simulink model "bi_real_unscr_4x_plan"  (Simulink 7.6)
settings: Solver=ode45  StartTime=0.0  StopTime=10.0  RelTol=1e-3
undefined symbols (not defined in the file or in its folder): add_latency
libraries: xbsIndex_r4 x259, casper_library x9, monroe_library x3
(part 1 of 2)
settings Model: Creator=monroe  LastModifiedBy=Ryan

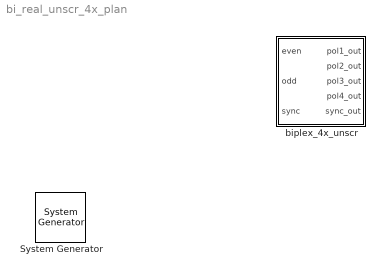
== system bi_real_unscr_4x_plan ==
  " System Generator" : xbsIndex_r4/ System Generator  Tag=genX  SystemSampleTime=-1  xilinxfamily=Virtex6  part=xc6vsx315t  speed=-3  package=ff1156  synthesis_tool=XST  clock_wrapper=Clock Enables  directory=./netlist  testbench=off  simulink_period=1  sysclk_period=10  dcm_input_clock_period=10  incr_netlist=off  trim_vbits=Everywhere in SubSystem  dbl_ovrd=According to Block Masks  core_generation=According to Block Masks  run_coregen=off  deprecated_control=off  eval_field=0  block_type=sysgen
  biplex_4x_unscr : Subsystem  mask{FFTSize=10, bram_latency=3, input_bit_width=18, reorder_din_latency=0}
      mask prompts: FFTSize "Size of FFT (2^?):"; bram_latency "BRAM Latency"; input_bit_width "Input Bit Width"; reorder_din_latency "Reorder Data In Latency"

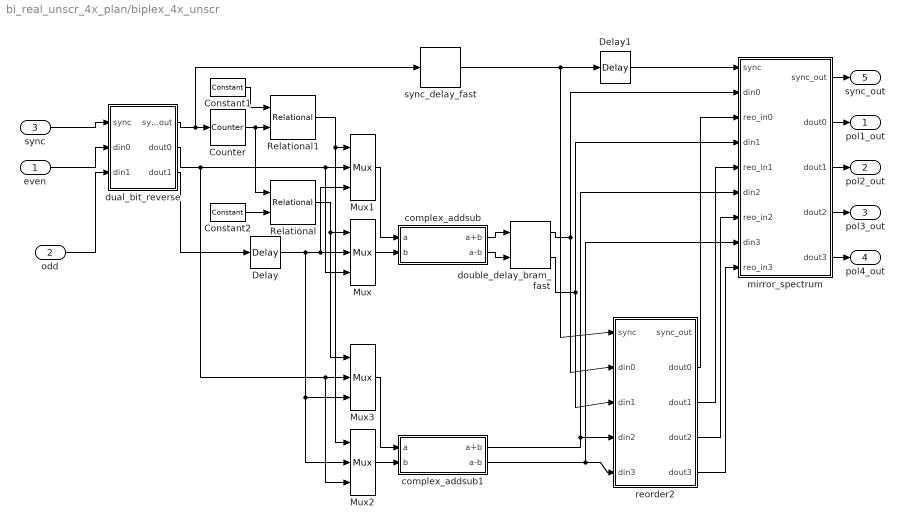
== system bi_real_unscr_4x_plan/biplex_4x_unscr ==
  even : Inport
  odd : Inport  Port=2
  sync : Inport  Port=3
  Constant1 : xbsIndex_r4/Constant  arith_type=Unsigned  const=2^(FFTSize-1)-1  n_bits=FFTSize  bin_pt=0  explicit_period=on  period=1  equ=P=C  opselect=C  inp2=PCIN>>17  opr=+  inp1=P  carry=CIN  dbl_ovrd=off  block_type=constant
      settings: block_version=9.1.01
  Constant2 : xbsIndex_r4/Constant  arith_type=Unsigned  const=2^FFTSize -1  n_bits=FFTSize  bin_pt=0  explicit_period=on  period=1  equ=P=C  opselect=C  inp2=PCIN>>17  opr=+  inp1=P  carry=CIN  dbl_ovrd=off  block_type=constant
      settings: block_version=9.1.01
  Counter : xbsIndex_r4/Counter  cnt_type=Free Running  cnt_to=Inf  operation=Up  start_count=0  cnt_by_val=1  arith_type=Unsigned  n_bits=FFTSize  bin_pt=0  load_pin=off  rst=on  en=off  explicit_period=off  period=1  dbl_ovrd=off  use_behavioral_HDL=off  implementation=Fabric  use_rpm=on  block_type=counter
      settings: xl_area=[0, 0, 0, 0, 0, 0, 0]  block_version=9.1.01
  Delay : xbsIndex_r4/Delay  en=off  latency=1  dbl_ovrd=off  reg_retiming=off  block_type=delay
      settings: xl_area=[0, 0, 0, 0, 0, 0, 0]  block_version=9.1.01
  Delay1 : xbsIndex_r4/Delay  en=off  latency=3  dbl_ovrd=off  reg_retiming=off  block_type=delay
      settings: xl_area=[0, 0, 0, 0, 0, 0, 0]  block_version=9.1.01
  Mux{,1..3} (4 alike) : xbsIndex_r4/Mux  inputs=2  en=off  latency=1  precision=Full  arith_type="Signed  (2's comp)"  n_bits=8  bin_pt=2  quantization=Truncate  overflow=Wrap  dbl_ovrd=off  block_type=mux
      settings: xl_area=[0, 0, 0, 0, 0, 0, 0]  block_version=9.1.01
  Relational : xbsIndex_r4/Relational  mode=a=b  en=off  latency=1  dbl_ovrd=off  block_type=relational
      settings: xl_area=[0, 0, 0, 0, 0, 0, 0]  block_version=9.1.01
  Relational1 : xbsIndex_r4/Relational  mode=a=b  en=off  latency=1  dbl_ovrd=off  block_type=relational
      settings: xl_area=[0, 0, 0, 0, 0, 0, 0]  block_version=9.1.01
  complex_addsub : Subsystem  mask(complex_addsub){BitWidth=input_bit_width, add_latency=add_latency}
      mask prompts: BitWidth "Bit Wdith"; add_latency "Add Latency"
      mask help:
      | Adds and subtracts the complex inputs.
      | If a = w + ix, b = y + iz then
      | a+b = (w+y)/2 + i(x-z)/2 and
      | a-b = (x+z)/2 + i(y-w)/2
  complex_addsub1 : Subsystem  mask(complex_addsub){BitWidth=input_bit_width, add_latency=add_latency}
      mask prompts: BitWidth "Bit Wdith"; add_latency "Add Latency"
      mask help:
      | Adds and subtracts the complex inputs.
      | If a = w + ix, b = y + iz then
      | a+b = (w+y)/2 + i(x-z)/2 and
      | a-b = (x+z)/2 + i(y-w)/2
  double_delay_bram_fast : monroe_library/double_delay_bram_fast  SystemSampleTime=-1  delay_len=2^(FFTSize-1)  bram_latency=bram_latency
  dual_bit_reverse : Subsystem  AncestorBlock=casper_library/Reorder/reorder  mask(reorder){bram_latency=bram_latency, din_latency=reorder_din_latency}
      mask prompts: bram_latency "BRAM Latency"; din_latency "Data In Latency"
      settings: AttributesFormatString=order=2
  mirror_spectrum : Subsystem
  reorder2 : Subsystem  AncestorBlock=casper_library/Reorder/reorder  mask(reorder){bram_latency=bram_latency, din_delay=1, map_latency=0, din_bit_width=input_bit_width}
      mask prompts: bram_latency "BRAM Latency"; din_delay "Data In Delay"; map_latency "Map Latency"; din_bit_width "Data In Bit Width"
      settings: AttributesFormatString=order=2
  sync_delay_fast : monroe_library/sync_delay_fast  SystemSampleTime=-1  delay_len=2^(FFTSize-1)+2
  pol1_out : Outport
  pol2_out : Outport  Port=2
  pol3_out : Outport  Port=3
  pol4_out : Outport  Port=4
  sync_out : Outport  Port=5
  wires:
  Delay1/1 -> mirror_spectrum/1(sync)
  mirror_spectrum/5(dout3) -> pol4_out/1
  mirror_spectrum/4(dout2) -> pol3_out/1
  mirror_spectrum/3(dout1) -> pol2_out/1
  odd/1 -> dual_bit_reverse/3(din1)
  even/1 -> dual_bit_reverse/2(din0)
  Relational/1 -> Mux3/1, Mux/1
  Mux/1 -> complex_addsub/2(b)
  Delay/1 -> Mux2/2, Mux3/3, Mux/2, Mux1/3
  dual_bit_reverse/1(sync_out) -> Counter/1, sync_delay_fast/1
  dual_bit_reverse/2(dout0) -> Mux/3, Mux1/2, Mux2/3, Mux3/2
  dual_bit_reverse/3(dout1) -> Delay/1
  sync/1 -> dual_bit_reverse/1(sync)
  Mux1/1 -> complex_addsub/1(a)
  Constant2/1 -> Relational/2
  Counter/1 -> Relational/1, Relational1/2
  Constant1/1 -> Relational1/1
  Relational1/1 -> Mux2/1, Mux1/1
  Mux2/1 -> complex_addsub1/2(b)
  Mux3/1 -> complex_addsub1/1(a)
  complex_addsub/1(a+b) -> double_delay_bram_fast/1
  complex_addsub/2(a-b) -> double_delay_bram_fast/2
  complex_addsub1/2(a-b) -> reorder2/5(din3), mirror_spectrum/8(din3)
  complex_addsub1/1(a+b) -> reorder2/4(din2), mirror_spectrum/6(din2)
  double_delay_bram_fast/2 -> reorder2/3(din1), mirror_spectrum/4(din1)
  double_delay_bram_fast/1 -> reorder2/2(din0), mirror_spectrum/2(din0)
  sync_delay_fast/1 -> Delay1/1, reorder2/1(sync)
  mirror_spectrum/1(sync_out) -> sync_out/1
  mirror_spectrum/2(dout0) -> pol1_out/1
  reorder2/3(dout1) -> mirror_spectrum/5(reo_in1)
  reorder2/2(dout0) -> mirror_spectrum/3(reo_in0)
  reorder2/4(dout2) -> mirror_spectrum/7(reo_in2)
  reorder2/5(dout3) -> mirror_spectrum/9(reo_in3)

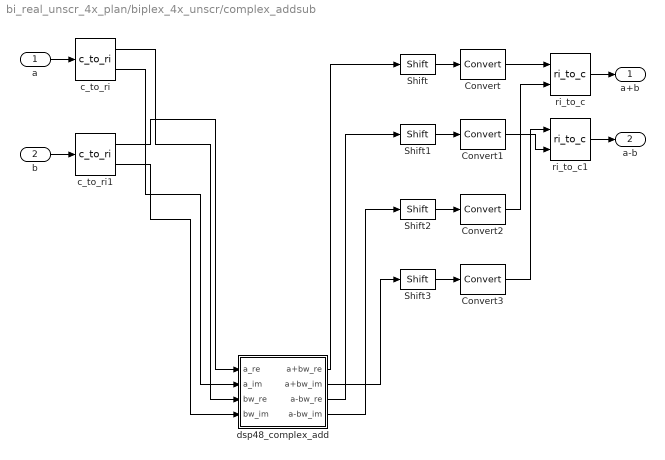
== system bi_real_unscr_4x_plan/biplex_4x_unscr/complex_addsub ==
  a : Inport
  b : Inport  Port=2
  Convert{,1..3} (4 alike) : xbsIndex_r4/Convert  arith_type="Signed  (2's comp)"  n_bits=BitWidth  bin_pt=BitWidth - 1  quantization=Truncate  overflow=Wrap  en=off  latency=add_latency  dbl_ovrd=off  pipeline=off  block_type=convert
      settings: xl_area=[0, 0, 0, 0, 0, 0, 0]
  Shift{,1..3} (4 alike) : xbsIndex_r4/Shift  shift_dir=Right  shift_bits=1  en=off  latency=0  precision=Full  arith_type="Signed  (2's comp)"  n_bits=8  bin_pt=2  quantization=Truncate  overflow=Wrap  dbl_ovrd=off  block_type=shift
      settings: xl_area=[0, 0, 0, 0, 0, 0, 0]  block_version=9.1.01
  c_to_ri : casper_library/Misc/c_to_ri  SystemSampleTime=-1  n_bits=BitWidth  bin_pt=BitWidth-1
      settings: AttributesFormatString=18_17 r/i
  c_to_ri1 : casper_library/Misc/c_to_ri  SystemSampleTime=-1  n_bits=BitWidth  bin_pt=BitWidth-1
      settings: AttributesFormatString=18_17 r/i
  dsp48_complex_add : Subsystem  mask{a_bit_width=BitWidth, a_bin_pt=BitWidth-2, bw_bit_width=BitWidth, bw_bin_pt=BitWidth-2}
      mask prompts: a_bit_width "'a' bit width"; a_bin_pt "'a' binary point"; bw_bit_width "'bw' bit width"; bw_bin_pt "'bw' binary point"
  ri_to_c : casper_library/Misc/ri_to_c  SystemSampleTime=-1
  ri_to_c1 : casper_library/Misc/ri_to_c  SystemSampleTime=-1
  a+b : Outport
  a-b : Outport  Port=2
  wires:
  Convert3/1 -> ri_to_c1/1
  Convert1/1 -> ri_to_c1/2
  c_to_ri/1 -> dsp48_complex_add/3(bw_re)
  c_to_ri/2 -> dsp48_complex_add/2(a_im)
  c_to_ri1/1 -> dsp48_complex_add/1(a_re)
  c_to_ri1/2 -> dsp48_complex_add/4(bw_im)
  Convert/1 -> ri_to_c/1
  Convert2/1 -> ri_to_c/2
  a/1 -> c_to_ri/1
  ri_to_c/1 -> a+b/1
  ri_to_c1/1 -> a-b/1
  b/1 -> c_to_ri1/1
  Shift/1 -> Convert/1
  Shift1/1 -> Convert1/1
  Shift2/1 -> Convert2/1
  Shift3/1 -> Convert3/1
  dsp48_complex_add/3(a-bw_re) -> Shift1/1
  dsp48_complex_add/4(a-bw_im) -> Shift2/1
  dsp48_complex_add/2(a+bw_im) -> Shift3/1
  dsp48_complex_add/1(a+bw_re) -> Shift/1

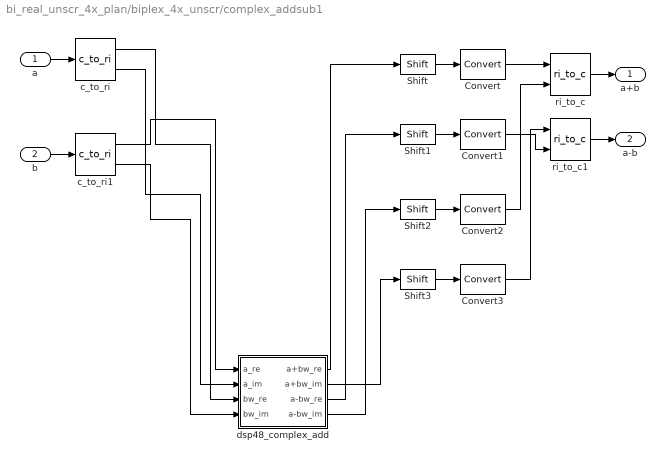
== system bi_real_unscr_4x_plan/biplex_4x_unscr/complex_addsub1 ==
  a : Inport
  b : Inport  Port=2
  Convert{,1..3} (4 alike) : xbsIndex_r4/Convert  arith_type="Signed  (2's comp)"  n_bits=BitWidth  bin_pt=BitWidth - 1  quantization=Truncate  overflow=Wrap  en=off  latency=add_latency  dbl_ovrd=off  pipeline=off  block_type=convert
      settings: xl_area=[0, 0, 0, 0, 0, 0, 0]
  Shift{,1..3} (4 alike) : xbsIndex_r4/Shift  shift_dir=Right  shift_bits=1  en=off  latency=0  precision=Full  arith_type="Signed  (2's comp)"  n_bits=8  bin_pt=2  quantization=Truncate  overflow=Wrap  dbl_ovrd=off  block_type=shift
      settings: xl_area=[0, 0, 0, 0, 0, 0, 0]  block_version=9.1.01
  c_to_ri : casper_library/Misc/c_to_ri  SystemSampleTime=-1  n_bits=BitWidth  bin_pt=BitWidth-1
      settings: AttributesFormatString=18_17 r/i
  c_to_ri1 : casper_library/Misc/c_to_ri  SystemSampleTime=-1  n_bits=BitWidth  bin_pt=BitWidth-1
      settings: AttributesFormatString=18_17 r/i
  dsp48_complex_add : Subsystem  mask{a_bit_width=BitWidth, a_bin_pt=BitWidth-2, bw_bit_width=BitWidth, bw_bin_pt=BitWidth-2}
      mask prompts: a_bit_width "'a' bit width"; a_bin_pt "'a' binary point"; bw_bit_width "'bw' bit width"; bw_bin_pt "'bw' binary point"
  ri_to_c : casper_library/Misc/ri_to_c  SystemSampleTime=-1
  ri_to_c1 : casper_library/Misc/ri_to_c  SystemSampleTime=-1
  a+b : Outport
  a-b : Outport  Port=2
  wires:
  dsp48_complex_add/1(a+bw_re) -> Shift/1
  dsp48_complex_add/2(a+bw_im) -> Shift3/1
  dsp48_complex_add/4(a-bw_im) -> Shift2/1
  dsp48_complex_add/3(a-bw_re) -> Shift1/1
  Shift3/1 -> Convert3/1
  Shift2/1 -> Convert2/1
  Shift1/1 -> Convert1/1
  Shift/1 -> Convert/1
  b/1 -> c_to_ri1/1
  ri_to_c1/1 -> a-b/1
  ri_to_c/1 -> a+b/1
  a/1 -> c_to_ri/1
  Convert2/1 -> ri_to_c/2
  Convert/1 -> ri_to_c/1
  c_to_ri1/2 -> dsp48_complex_add/4(bw_im)
  c_to_ri1/1 -> dsp48_complex_add/1(a_re)
  c_to_ri/2 -> dsp48_complex_add/2(a_im)
  c_to_ri/1 -> dsp48_complex_add/3(bw_re)
  Convert1/1 -> ri_to_c1/2
  Convert3/1 -> ri_to_c1/1

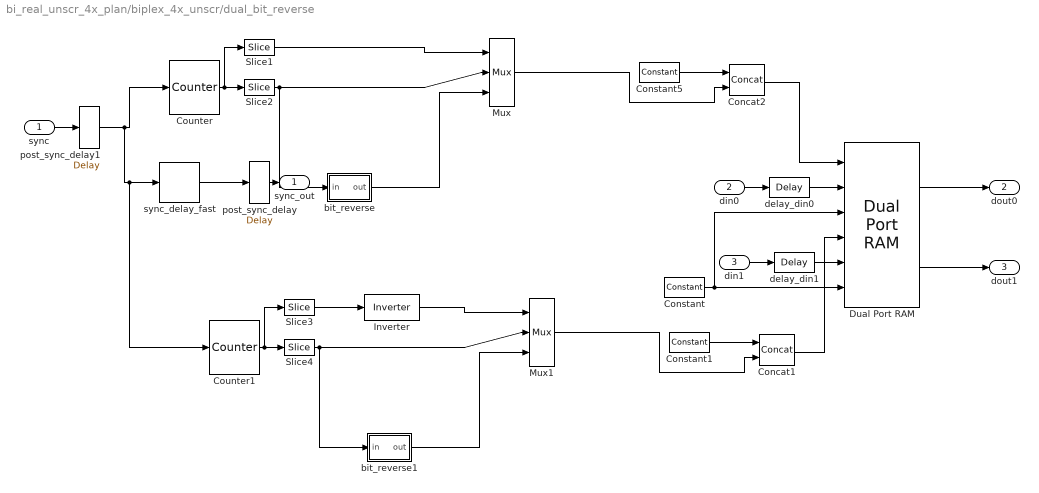
== system bi_real_unscr_4x_plan/biplex_4x_unscr/dual_bit_reverse ==
  sync : Inport
  din0 : Inport  Port=2
  din1 : Inport  Port=3
  Concat1 : xbsIndex_r4/Concat  num_inputs=2  dbl_ovrd=off  block_type=concat
  Concat2 : xbsIndex_r4/Concat  num_inputs=2  dbl_ovrd=off  block_type=concat
  Constant : xbsIndex_r4/Constant  arith_type=Boolean  const=1  n_bits=1  bin_pt=0  explicit_period=on  period=1  equ=P=C  opselect=C  inp2=PCIN>>17  opr=+  inp1=P  carry=CIN  dbl_ovrd=off  block_type=constant
      settings: block_version=9.1.01
  Constant1 : xbsIndex_r4/Constant  arith_type=Boolean  const=0  n_bits=1  bin_pt=0  explicit_period=on  period=1  equ=P=C  opselect=C  inp2=PCIN>>17  opr=+  inp1=P  carry=CIN  dbl_ovrd=off  block_type=constant
      settings: block_version=9.1.01
  Constant5 : xbsIndex_r4/Constant  arith_type=Boolean  const=1  n_bits=1  bin_pt=0  explicit_period=on  period=1  equ=P=C  opselect=C  inp2=PCIN>>17  opr=+  inp1=P  carry=CIN  dbl_ovrd=off  block_type=constant
      settings: block_version=9.1.01
  Counter : xbsIndex_r4/Counter  cnt_type=Free Running  cnt_to=1023  operation=Up  start_count=0  cnt_by_val=1  arith_type=Unsigned  n_bits=FFTSize  bin_pt=0  load_pin=off  rst=on  en=off  explicit_period=on  period=1  dbl_ovrd=off  use_behavioral_HDL=off  implementation=Fabric  use_rpm=off  block_type=counter
  Counter1 : xbsIndex_r4/Counter  cnt_type=Free Running  cnt_to=1023  operation=Down  start_count=(2^FFTSize)-1  cnt_by_val=1  arith_type=Unsigned  n_bits=FFTSize  bin_pt=0  load_pin=off  rst=on  en=off  explicit_period=on  period=1  dbl_ovrd=off  use_behavioral_HDL=off  implementation=Fabric  use_rpm=off  block_type=counter
  Dual Port RAM : xbsIndex_r4/Dual Port RAM  depth=2^(FFTSize)  initVector=sin(pi*(0:15)/16)  distributed_mem=Block RAM  init_a=0  init_b=0  rst_a=off  rst_b=off  en_a=off  en_b=off  latency=bram_latency  write_mode_A=Read Before Write  write_mode_B=Read Before Write  dbl_ovrd=off  optimize=Area  use_rpm=on  block_type=dpram
  Inverter : xbsIndex_r4/Inverter  en=off  latency=0  dbl_ovrd=off  block_type=inv
  Mux : xbsIndex_r4/Mux  inputs=2  en=off  latency=0  precision=Full  arith_type=Unsigned  n_bits=16  bin_pt=14  quantization=Truncate  overflow=Wrap  dbl_ovrd=off  block_type=mux
  Mux1 : xbsIndex_r4/Mux  inputs=2  en=off  latency=0  precision=Full  arith_type=Unsigned  n_bits=16  bin_pt=14  quantization=Truncate  overflow=Wrap  dbl_ovrd=off  block_type=mux
  Slice1 : xbsIndex_r4/Slice  nbits=1  boolean_output=off  mode=Upper Bit Location + Width  bit1=0  base1=MSB of Input  bit0=0  base0=LSB of Input  dbl_ovrd=off  block_type=slice
      settings: infoedit="Extracts a given range of bits from each input sample and presents it at the output.  The output type is ordinarily unsigned with binary point at zero, but can be Boolean when the slice is one bit wide.<P><P>Hardware notes: In hardware this block costs nothing."  block_version=10.1.3
  Slice2 : xbsIndex_r4/Slice  nbits=FFTSize-1  boolean_output=off  mode=Lower Bit Location + Width  bit1=0  base1=MSB of Input  bit0=0  base0=LSB of Input  dbl_ovrd=off  block_type=slice
      settings: block_version=10.1.3
  Slice3 : xbsIndex_r4/Slice  nbits=1  boolean_output=off  mode=Upper Bit Location + Width  bit1=0  base1=MSB of Input  bit0=0  base0=LSB of Input  dbl_ovrd=off  block_type=slice
      settings: infoedit="Extracts a given range of bits from each input sample and presents it at the output.  The output type is ordinarily unsigned with binary point at zero, but can be Boolean when the slice is one bit wide.<P><P>Hardware notes: In hardware this block costs nothing."  block_version=10.1.3
  Slice4 : xbsIndex_r4/Slice  nbits=FFTSize-1  boolean_output=off  mode=Lower Bit Location + Width  bit1=0  base1=MSB of Input  bit0=0  base0=LSB of Input  dbl_ovrd=off  block_type=slice
      settings: block_version=10.1.3
  bit_reverse : Subsystem  mask{nBits=FFTSize-1}
      mask prompts: nBits "# bits?"
      mask init:
      | config.source=str2func('bit_reverse_draw');
      | config.toplevel=gcb;
      | config.debug=0;
      | config.depend={'bit_reverse_draw.m'};
      | %xBlock(config,{nBits,1});
  bit_reverse1 : Subsystem  mask{nBits=FFTSize-1}
      mask prompts: nBits "# bits?"
      mask init:
      | config.source=str2func('bit_reverse_draw');
      | config.toplevel=gcb;
      | config.debug=0;
      | config.depend={'bit_reverse_draw.m'};
      | %xBlock(config,{nBits,1});
  delay_din0 : xbsIndex_r4/Delay  en=off  latency=din_latency  dbl_ovrd=off  reg_retiming=off  block_type=delay
      settings: xl_area=[0, 0, 0, 0, 0, 0, 0]  block_version=9.1.01
  delay_din1 : xbsIndex_r4/Delay  en=off  latency=din_latency  dbl_ovrd=off  reg_retiming=off  block_type=delay
      settings: xl_area=[0, 0, 0, 0, 0, 0, 0]  block_version=9.1.01
  post_sync_delay : xbsIndex_r4/Delay  en=off  latency=bram_latency  dbl_ovrd=off  reg_retiming=off  block_type=delay
      settings: xl_area=[0, 0, 0, 0, 0, 0, 0]  block_version=9.1.01
  post_sync_delay1 : xbsIndex_r4/Delay  en=off  latency=din_latency  dbl_ovrd=off  reg_retiming=off  block_type=delay
      settings: xl_area=[0, 0, 0, 0, 0, 0, 0]  block_version=9.1.01
  sync_delay_fast : monroe_library/sync_delay_fast  SystemSampleTime=-1  delay_len=2^(FFTSize-1)
  sync_out : Outport
  dout0 : Outport  Port=2
  dout1 : Outport  Port=3
  wires:
  bit_reverse/1(out) -> Mux/3
  din0/1 -> delay_din0/1
  post_sync_delay/1 -> sync_out/1
  sync_delay_fast/1 -> post_sync_delay/1
  Slice2/1 -> Mux/2, bit_reverse/1(in)
  Slice1/1 -> Mux/1
  Counter/1 -> Slice1/1, Slice2/1
  Counter1/1 -> Slice4/1, Slice3/1
  Slice3/1 -> Inverter/1
  Slice4/1 -> bit_reverse1/1(in), Mux1/2
  din1/1 -> delay_din1/1
  bit_reverse1/1(out) -> Mux1/3
  Inverter/1 -> Mux1/1
  sync/1 -> post_sync_delay1/1
  post_sync_delay1/1 -> Counter/1, sync_delay_fast/1, Counter1/1
  delay_din0/1 -> Dual Port RAM/2
  delay_din1/1 -> Dual Port RAM/5
  Constant/1 -> Dual Port RAM/6, Dual Port RAM/3
  Dual Port RAM/1 -> dout0/1
  Dual Port RAM/2 -> dout1/1
  Constant5/1 -> Concat2/1
  Concat2/1 -> Dual Port RAM/1
  Mux/1 -> Concat2/2
  Constant1/1 -> Concat1/1
  Concat1/1 -> Dual Port RAM/4
  Mux1/1 -> Concat1/2

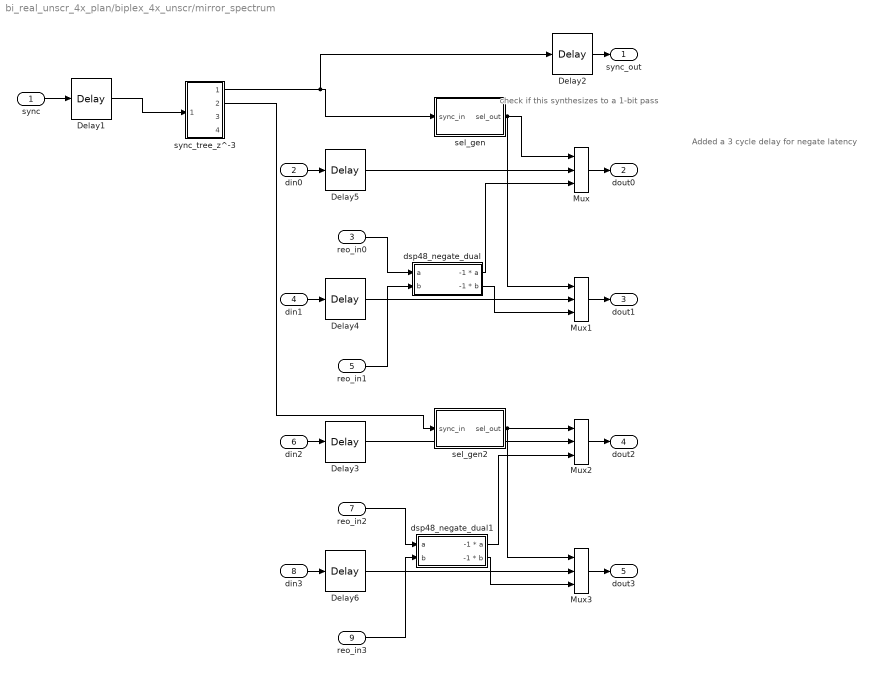
== system bi_real_unscr_4x_plan/biplex_4x_unscr/mirror_spectrum ==
  note: check if this synthesizes
      | to a 1-bit pass
  note: Added a 3 cycle delay for negate latency
  sync : Inport
  din0 : Inport  Port=2
  reo_in0 : Inport  Port=3
  din1 : Inport  Port=4
  reo_in1 : Inport  Port=5
  din2 : Inport  Port=6
  reo_in2 : Inport  Port=7
  din3 : Inport  Port=8
  reo_in3 : Inport  Port=9
  Delay1 : xbsIndex_r4/Delay  en=off  latency=2  dbl_ovrd=off  reg_retiming=off  block_type=delay
      settings: xl_area=[0, 0, 0, 0, 0, 0, 0]  block_version=9.1.01
  Delay2 : xbsIndex_r4/Delay  en=off  latency=1  dbl_ovrd=off  reg_retiming=off  block_type=delay
      settings: xl_area=[0, 0, 0, 0, 0, 0, 0]  block_version=9.1.01
  Delay{3..6} (4 alike) : xbsIndex_r4/Delay  en=off  latency=bram_latency - 1 + 1 + 3  dbl_ovrd=off  reg_retiming=off  block_type=delay
      settings: xl_area=[0, 0, 0, 0, 0, 0, 0]  block_version=9.1.01
  Mux{,1..3} (4 alike) : xbsIndex_r4/Mux  inputs=2  en=off  latency=0  precision=Full  arith_type="Signed  (2's comp)"  n_bits=8  bin_pt=2  quantization=Truncate  overflow=Wrap  dbl_ovrd=off  block_type=mux
      settings: xl_area=[0, 0, 0, 0, 0, 0, 0]  block_version=9.1.01
  dsp48_negate_dual : Subsystem  mask{a_bit_width=input_bit_width, a_bin_pt=input_bit_width-1}
      mask prompts: a_bit_width "bit width"; a_bin_pt "binary point"
  dsp48_negate_dual1 : Subsystem  mask{a_bit_width=input_bit_width, a_bin_pt=input_bit_width-1}
      mask prompts: a_bit_width "bit width"; a_bin_pt "binary point"
  sel_gen : Subsystem
  sel_gen2 : Subsystem
  sync_tree_z^-3 : Subsystem
  sync_out : Outport
  dout0 : Outport  Port=2
  dout1 : Outport  Port=3
  dout2 : Outport  Port=4
  dout3 : Outport  Port=5
  wires:
  sync_tree_z^-3/1(Out1) -> Delay2/1, sel_gen/1(sync_in)
  Delay1/1 -> sync_tree_z^-3/1(In1)
  sel_gen2/1(sel_out) -> Mux2/1, Mux3/1
  sel_gen/1(sel_out) -> Mux/1, Mux1/1
  din3/1 -> Delay6/1
  Delay6/1 -> Mux3/2
  Mux3/1 -> dout3/1
  reo_in3/1 -> dsp48_negate_dual1/2(b)
  dsp48_negate_dual1/2(-1 * b) -> Mux3/3
  din2/1 -> Delay3/1
  Delay3/1 -> Mux2/2
  Mux2/1 -> dout2/1
  reo_in2/1 -> dsp48_negate_dual1/1(a)
  dsp48_negate_dual1/1(-1 * a) -> Mux2/3
  din1/1 -> Delay4/1
  Delay4/1 -> Mux1/2
  Mux1/1 -> dout1/1
  reo_in1/1 -> dsp48_negate_dual/2(b)
  sync/1 -> Delay1/1
  din0/1 -> Delay5/1
  Delay5/1 -> Mux/2
  Mux/1 -> dout0/1
  Delay2/1 -> sync_out/1
  reo_in0/1 -> dsp48_negate_dual/1(a)
  dsp48_negate_dual/1(-1 * a) -> Mux/3
  sync_tree_z^-3/2(Out2) -> sel_gen2/1(sync_in)
  dsp48_negate_dual/2(-1 * b) -> Mux1/3

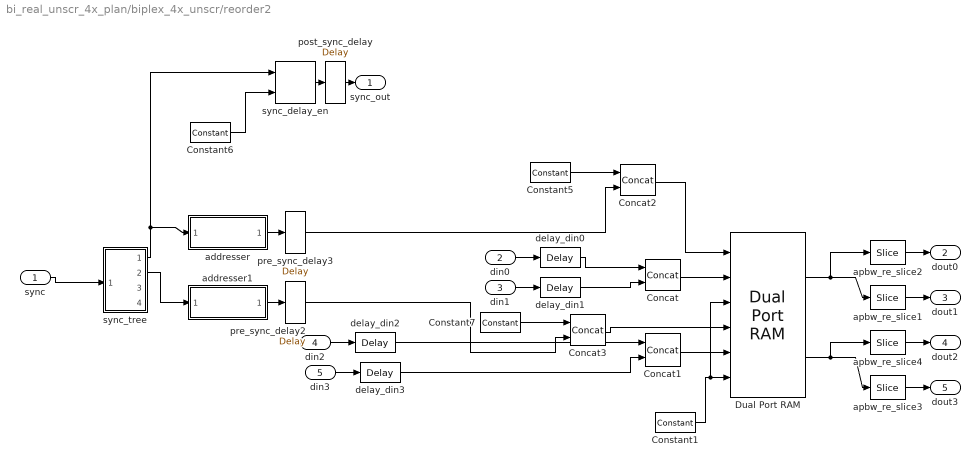
== system bi_real_unscr_4x_plan/biplex_4x_unscr/reorder2 ==
  sync : Inport
  din0 : Inport  Port=2
  din1 : Inport  Port=3
  din2 : Inport  Port=4
  din3 : Inport  Port=5
  Concat{,1..3} (4 alike) : xbsIndex_r4/Concat  num_inputs=2  dbl_ovrd=off  block_type=concat
  Constant1 : xbsIndex_r4/Constant  arith_type=Boolean  const=1  n_bits=1  bin_pt=0  explicit_period=on  period=1  equ=P=C  opselect=C  inp2=PCIN>>17  opr=+  inp1=P  carry=CIN  dbl_ovrd=off  block_type=constant
      settings: block_version=9.1.01
  Constant5 : xbsIndex_r4/Constant  arith_type=Boolean  const=1  n_bits=1  bin_pt=0  explicit_period=on  period=1  equ=P=C  opselect=C  inp2=PCIN>>17  opr=+  inp1=P  carry=CIN  dbl_ovrd=off  block_type=constant
      settings: block_version=9.1.01
  Constant6 : xbsIndex_r4/Constant  arith_type=Boolean  const=1  n_bits=1  bin_pt=0  explicit_period=on  period=1  equ=P=C  opselect=C  inp2=PCIN>>17  opr=+  inp1=P  carry=CIN  dbl_ovrd=off  block_type=constant
      settings: block_version=9.1.01
  Constant7 : xbsIndex_r4/Constant  arith_type=Boolean  const=0  n_bits=1  bin_pt=0  explicit_period=on  period=1  equ=P=C  opselect=C  inp2=PCIN>>17  opr=+  inp1=P  carry=CIN  dbl_ovrd=off  block_type=constant
      settings: block_version=9.1.01
  Dual Port RAM : xbsIndex_r4/Dual Port RAM  depth=2^(FFTSize+1)  initVector=sin(pi*(0:15)/16)  distributed_mem=Block RAM  init_a=0  init_b=0  rst_a=off  rst_b=off  en_a=off  en_b=off  latency=bram_latency  write_mode_A=Read Before Write  write_mode_B=Read Before Write  dbl_ovrd=off  optimize=Area  use_rpm=on  block_type=dpram
  addresser : Subsystem
  addresser1 : Subsystem
  apbw_re_slice1 : xbsIndex_r4/Slice  nbits=din_bit_width*2  boolean_output=off  mode=Lower Bit Location + Width  bit1=0  base1=MSB of Input  bit0=0  base0=LSB of Input  dbl_ovrd=off  block_type=slice
      settings: block_version=11.3
  apbw_re_slice2 : xbsIndex_r4/Slice  nbits=din_bit_width*2  boolean_output=off  mode=Lower Bit Location + Width  bit1=0  base1=MSB of Input  bit0=din_bit_width*2  base0=LSB of Input  dbl_ovrd=off  block_type=slice
      settings: block_version=11.3
  apbw_re_slice3 : xbsIndex_r4/Slice  nbits=din_bit_width*2  boolean_output=off  mode=Lower Bit Location + Width  bit1=0  base1=MSB of Input  bit0=0  base0=LSB of Input  dbl_ovrd=off  block_type=slice
      settings: block_version=11.3
  apbw_re_slice4 : xbsIndex_r4/Slice  nbits=din_bit_width*2  boolean_output=off  mode=Lower Bit Location + Width  bit1=0  base1=MSB of Input  bit0=din_bit_width*2  base0=LSB of Input  dbl_ovrd=off  block_type=slice
      settings: block_version=11.3
  delay_din{0..3} (4 alike) : xbsIndex_r4/Delay  en=off  latency=din_delay  dbl_ovrd=off  reg_retiming=off  block_type=delay
      settings: xl_area=[0, 0, 0, 0, 0, 0, 0]  block_version=9.1.01
  post_sync_delay : xbsIndex_r4/Delay  en=off  latency=3+din_delay+map_latency  dbl_ovrd=off  reg_retiming=off  block_type=delay
      settings: xl_area=[0, 0, 0, 0, 0, 0, 0]  block_version=9.1.01
  pre_sync_delay2 : xbsIndex_r4/Delay  en=off  latency=din_delay  dbl_ovrd=off  reg_retiming=off  block_type=delay
      settings: xl_area=[0, 0, 0, 0, 0, 0, 0]  block_version=9.1.01
  pre_sync_delay3 : xbsIndex_r4/Delay  en=off  latency=din_delay  dbl_ovrd=off  reg_retiming=off  block_type=delay
      settings: xl_area=[0, 0, 0, 0, 0, 0, 0]  block_version=9.1.01
  sync_delay_en : casper_library/Delays/sync_delay_en  SystemSampleTime=-1  DelayLen=512
  sync_tree : Subsystem
  sync_out : Outport
  dout0 : Outport  Port=2
  dout1 : Outport  Port=3
  dout2 : Outport  Port=4
  dout3 : Outport  Port=5
  wires:
  sync_tree/2(Out2) -> addresser1/1(sync_in)
  sync_tree/1(Out1) -> addresser/1(sync_in), sync_delay_en/1
  Constant6/1 -> sync_delay_en/2
  delay_din3/1 -> Concat1/2
  din3/1 -> delay_din3/1
  din2/1 -> delay_din2/1
  apbw_re_slice1/1 -> dout1/1
  delay_din1/1 -> Concat/2
  din1/1 -> delay_din1/1
  apbw_re_slice2/1 -> dout0/1
  delay_din0/1 -> Concat/1
  din0/1 -> delay_din0/1
  post_sync_delay/1 -> sync_out/1
  sync_delay_en/1 -> post_sync_delay/1
  Constant1/1 -> Dual Port RAM/6, Dual Port RAM/3
  sync/1 -> sync_tree/1(In1)
  addresser1/1(addr_out) -> pre_sync_delay2/1
  addresser/1(addr_out) -> pre_sync_delay3/1
  Concat/1 -> Dual Port RAM/2
  Concat1/1 -> Dual Port RAM/5
  Constant5/1 -> Concat2/1
  Constant7/1 -> Concat3/1
  Concat3/1 -> Dual Port RAM/4
  Concat2/1 -> Dual Port RAM/1
  delay_din2/1 -> Concat1/1
  pre_sync_delay2/1 -> Concat3/2
  apbw_re_slice4/1 -> dout2/1
  apbw_re_slice3/1 -> dout3/1
  Dual Port RAM/1 -> apbw_re_slice2/1, apbw_re_slice1/1
  Dual Port RAM/2 -> apbw_re_slice4/1, apbw_re_slice3/1
  pre_sync_delay3/1 -> Concat2/2

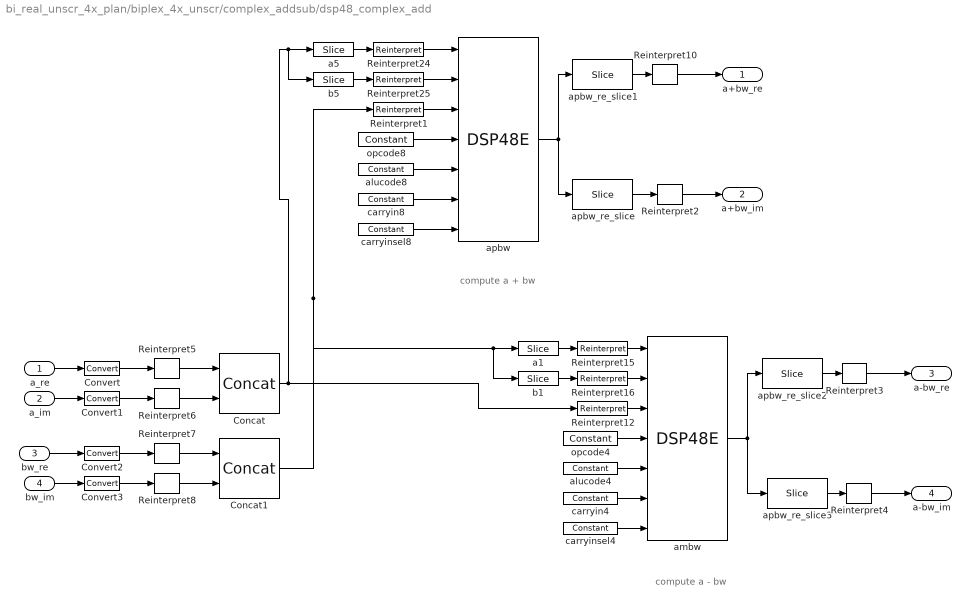
== system bi_real_unscr_4x_plan/biplex_4x_unscr/complex_addsub/dsp48_complex_add ==
  note: compute a + bw
  note: compute a - bw
  a_re : Inport
  a_im : Inport  Port=2
  bw_re : Inport  Port=3
  bw_im : Inport  Port=4
  Concat : xbsIndex_r4/Concat  num_inputs=2  dbl_ovrd=off  block_type=concat
      settings: block_version=11.3
  Concat1 : xbsIndex_r4/Concat  num_inputs=2  dbl_ovrd=off  block_type=concat
      settings: block_version=11.3
  Convert{,1..3} (4 alike) : xbsIndex_r4/Convert  arith_type="Signed  (2's comp)"  n_bits=24  bin_pt=24 - (bw_bit_width - bw_bin_pt)  quantization=Truncate  overflow=Wrap  en=off  latency=0  dbl_ovrd=off  pipeline=off  block_type=convert
      settings: block_version=11.4
  Reinterpret{1,12,15..16,24..25} (6 alike) : xbsIndex_r4/Reinterpret  force_arith_type=on  arith_type="Signed  (2's comp)"  force_bin_pt=off  bin_pt=0  block_type=reinterpret
      settings: infoedit="Changes signal type without altering the binary representation.   You can changed the signal between signed and unsigned, and relocate the binary point.<br><br>Hardware notes: In hardware this block costs nothing.<br><br>Example:  Suppose the input is 6 bits wide, signed, with 2 fractional bits, and the output is forced to unsigned with 0 fractional bits.  Then an input of -2.0 (1110.00 in binary 2's complement) becomes an output of 56 (111000 in binary)."  block_version=11.3
  Reinterpret{2..4,10} (4 alike) : xbsIndex_r4/Reinterpret  force_arith_type=on  arith_type="Signed  (2's comp)"  force_bin_pt=on  bin_pt=24 - (bw_bit_width - bw_bin_pt)  block_type=reinterpret
      settings: infoedit="Changes signal type without altering the binary representation.   You can changed the signal between signed and unsigned, and relocate the binary point.<br><br>Hardware notes: In hardware this block costs nothing.<br><br>Example:  Suppose the input is 6 bits wide, signed, with 2 fractional bits, and the output is forced to unsigned with 0 fractional bits.  Then an input of -2.0 (1110.00 in binary 2's complement) becomes an output of 56 (111000 in binary)."  block_version=11.3
  Reinterpret{5..8} (4 alike) : xbsIndex_r4/Reinterpret  force_arith_type=on  arith_type=Unsigned  force_bin_pt=on  bin_pt=0  block_type=reinterpret
      settings: infoedit="Changes signal type without altering the binary representation.   You can changed the signal between signed and unsigned, and relocate the binary point.<br><br>Hardware notes: In hardware this block costs nothing.<br><br>Example:  Suppose the input is 6 bits wide, signed, with 2 fractional bits, and the output is forced to unsigned with 0 fractional bits.  Then an input of -2.0 (1110.00 in binary 2's complement) becomes an output of 56 (111000 in binary)."  block_version=11.3
  a1 : xbsIndex_r4/Slice  nbits=30  boolean_output=off  mode=Upper Bit Location + Width  bit1=0  base1=MSB of Input  bit0=18  base0=LSB of Input  dbl_ovrd=off  block_type=slice
      settings: block_version=11.3
  a5 : xbsIndex_r4/Slice  nbits=30  boolean_output=off  mode=Upper Bit Location + Width  bit1=0  base1=MSB of Input  bit0=18  base0=LSB of Input  dbl_ovrd=off  block_type=slice
      settings: block_version=11.3
  alucode4 : xbsIndex_r4/Constant  arith_type=Unsigned  const=3  n_bits=4  bin_pt=0  explicit_period=on  period=1  equ=P=C  opselect=C  inp2=PCIN>>17  opr=+  inp1=P  carry=CIN  dbl_ovrd=off  block_type=constant
  alucode8 : xbsIndex_r4/Constant  arith_type=Unsigned  const=0  n_bits=4  bin_pt=0  explicit_period=on  period=1  equ=P=C  opselect=C  inp2=PCIN>>17  opr=+  inp1=P  carry=CIN  dbl_ovrd=off  block_type=constant
  ambw : xbsIndex_r4/DSP48E  use_a=Direct from A Port  use_b=Direct from B Port  reset_preg=off  pattern_from_creg=off  pattern='000000000000'  mask_from_creg=off  pattern_mask='3FFFFFFFFFFF'  sel_rounding_mask=Select mask  use_op=off  use_creg=on  rst_all=off  en_all=off  use_pcin=off  use_carrycascin=off  use_multsignin=off  use_carryout=off  use_patterndetect=off  use_patternbdetect=off  use_overflow=off  use_underflow=off  use_acout=off  use_bcout=off  use_pcout=off  use_multsignout=off  use_carrycascout=off  pipeline_a=1  pipeline_b=1  pipeline_acout=1  pipeline_bcout=1  pipeline_c=on  pipeline_p=on  pipeline_mult=on  pipeline_opmode=on  pipeline_alumode=on  pipeline_carryin=on  pipeline_carryinsel=on  rst_a=off  rst_b=off  rst_c=off  rst_mult=off  rst_p=off  rst_carry_in=off  rst_alumode=off  rst_ctrl=off  en_a1=off  en_a2=off  en_b1=off  en_b2=off  en_c=off  en_mult=off  en_p=off  en_carry_in=off  en_alumode=off  en_multcarryin=off  en_ctrl=off  use_synth_model=off  addsub_mode=TWO24  xl_useadderonly=off  block_type=dsp48e
      settings: block_version=10.1.3
  apbw : xbsIndex_r4/DSP48E  use_a=Direct from A Port  use_b=Direct from B Port  reset_preg=off  pattern_from_creg=off  pattern='000000000000'  mask_from_creg=off  pattern_mask='3FFFFFFFFFFF'  sel_rounding_mask=Select mask  use_op=off  use_creg=on  rst_all=off  en_all=off  use_pcin=off  use_carrycascin=off  use_multsignin=off  use_carryout=off  use_patterndetect=off  use_patternbdetect=off  use_overflow=off  use_underflow=off  use_acout=off  use_bcout=off  use_pcout=off  use_multsignout=off  use_carrycascout=off  pipeline_a=1  pipeline_b=1  pipeline_acout=1  pipeline_bcout=1  pipeline_c=on  pipeline_p=on  pipeline_mult=on  pipeline_opmode=on  pipeline_alumode=on  pipeline_carryin=on  pipeline_carryinsel=on  rst_a=off  rst_b=off  rst_c=off  rst_mult=off  rst_p=off  rst_carry_in=off  rst_alumode=off  rst_ctrl=off  en_a1=off  en_a2=off  en_b1=off  en_b2=off  en_c=off  en_mult=off  en_p=off  en_carry_in=off  en_alumode=off  en_multcarryin=off  en_ctrl=off  use_synth_model=off  addsub_mode=TWO24  xl_useadderonly=off  block_type=dsp48e
      settings: block_version=10.1.3
  apbw_re_slice : xbsIndex_r4/Slice  nbits=24  boolean_output=off  mode=Lower Bit Location + Width  bit1=0  base1=MSB of Input  bit0=0  base0=LSB of Input  dbl_ovrd=off  block_type=slice
      settings: block_version=11.3
  apbw_re_slice1 : xbsIndex_r4/Slice  nbits=24  boolean_output=off  mode=Upper Bit Location + Width  bit1=0  base1=MSB of Input  bit0=24  base0=LSB of Input  dbl_ovrd=off  block_type=slice
      settings: block_version=11.3
  apbw_re_slice2 : xbsIndex_r4/Slice  nbits=24  boolean_output=off  mode=Upper Bit Location + Width  bit1=0  base1=MSB of Input  bit0=24  base0=LSB of Input  dbl_ovrd=off  block_type=slice
      settings: block_version=11.3
  apbw_re_slice3 : xbsIndex_r4/Slice  nbits=24  boolean_output=off  mode=Lower Bit Location + Width  bit1=0  base1=MSB of Input  bit0=0  base0=LSB of Input  dbl_ovrd=off  block_type=slice
      settings: block_version=11.3
  b1 : xbsIndex_r4/Slice  nbits=18  boolean_output=off  mode=Lower Bit Location + Width  bit1=0  base1=MSB of Input  bit0=0  base0=LSB of Input  dbl_ovrd=off  block_type=slice
      settings: block_version=11.3
  b5 : xbsIndex_r4/Slice  nbits=18  boolean_output=off  mode=Lower Bit Location + Width  bit1=0  base1=MSB of Input  bit0=0  base0=LSB of Input  dbl_ovrd=off  block_type=slice
      settings: block_version=11.3
  carryin4 : xbsIndex_r4/Constant  arith_type=Unsigned  const=0  n_bits=1  bin_pt=0  explicit_period=on  period=1  equ=P=C  opselect=C  inp2=PCIN>>17  opr=+  inp1=P  carry=CIN  dbl_ovrd=off  block_type=constant
  carryin8 : xbsIndex_r4/Constant  arith_type=Unsigned  const=0  n_bits=1  bin_pt=0  explicit_period=on  period=1  equ=P=C  opselect=C  inp2=PCIN>>17  opr=+  inp1=P  carry=CIN  dbl_ovrd=off  block_type=constant
  carryinsel4 : xbsIndex_r4/Constant  arith_type=Unsigned  const=0  n_bits=3  bin_pt=0  explicit_period=on  period=1  equ=P=C  opselect=C  inp2=PCIN>>17  opr=+  inp1=P  carry=CIN  dbl_ovrd=off  block_type=constant
  carryinsel8 : xbsIndex_r4/Constant  arith_type=Unsigned  const=0  n_bits=3  bin_pt=0  explicit_period=on  period=1  equ=P=C  opselect=C  inp2=PCIN>>17  opr=+  inp1=P  carry=CIN  dbl_ovrd=off  block_type=constant
  opcode4 : xbsIndex_r4/Constant  arith_type=Unsigned  const=51  n_bits=7  bin_pt=0  explicit_period=on  period=1  equ=P=C  opselect=C  inp2=PCIN>>17  opr=+  inp1=P  carry=CIN  dbl_ovrd=off  block_type=constant
  opcode8 : xbsIndex_r4/Constant  arith_type=Unsigned  const=15  n_bits=7  bin_pt=0  explicit_period=on  period=1  equ=P=C  opselect=C  inp2=PCIN>>17  opr=+  inp1=P  carry=CIN  dbl_ovrd=off  block_type=constant
  a+bw_re : Outport
  a+bw_im : Outport  Port=2
  a-bw_re : Outport  Port=3
  a-bw_im : Outport  Port=4
  wires:
  a_re/1 -> Convert/1
  a_im/1 -> Convert1/1
  bw_re/1 -> Convert2/1
  bw_im/1 -> Convert3/1
  Concat/1 -> Reinterpret12/1, a5/1, b5/1
  Concat1/1 -> Reinterpret1/1, b1/1, a1/1
  apbw_re_slice1/1 -> Reinterpret10/1
  a5/1 -> Reinterpret24/1
  Reinterpret24/1 -> apbw/1
  b5/1 -> Reinterpret25/1
  Reinterpret25/1 -> apbw/2
  opcode8/1 -> apbw/4
  alucode8/1 -> apbw/5
  carryin8/1 -> apbw/6
  carryinsel8/1 -> apbw/7
  apbw/1 -> apbw_re_slice/1, apbw_re_slice1/1
  apbw_re_slice/1 -> Reinterpret2/1
  Reinterpret1/1 -> apbw/3
  Reinterpret10/1 -> a+bw_re/1
  apbw_re_slice2/1 -> Reinterpret3/1
  a1/1 -> Reinterpret15/1
  Reinterpret15/1 -> ambw/1
  b1/1 -> Reinterpret16/1
  Reinterpret16/1 -> ambw/2
  opcode4/1 -> ambw/4
  alucode4/1 -> ambw/5
  carryin4/1 -> ambw/6
  carryinsel4/1 -> ambw/7
  ambw/1 -> apbw_re_slice3/1, apbw_re_slice2/1
  apbw_re_slice3/1 -> Reinterpret4/1
  Reinterpret12/1 -> ambw/3
  Reinterpret2/1 -> a+bw_im/1
  Reinterpret3/1 -> a-bw_re/1
  Reinterpret4/1 -> a-bw_im/1
  Convert/1 -> Reinterpret5/1
  Convert1/1 -> Reinterpret6/1
  Convert2/1 -> Reinterpret7/1
  Convert3/1 -> Reinterpret8/1
  Reinterpret5/1 -> Concat/1
  Reinterpret6/1 -> Concat/2
  Reinterpret7/1 -> Concat1/1
  Reinterpret8/1 -> Concat1/2

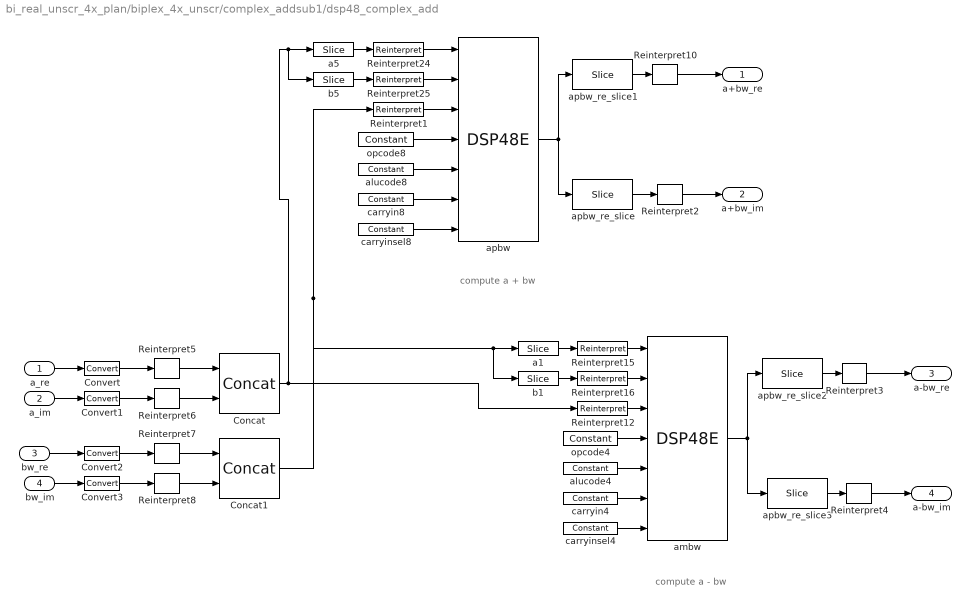
== system bi_real_unscr_4x_plan/biplex_4x_unscr/complex_addsub1/dsp48_complex_add ==
  note: compute a - bw
  note: compute a + bw
  a_re : Inport
  a_im : Inport  Port=2
  bw_re : Inport  Port=3
  bw_im : Inport  Port=4
  Concat : xbsIndex_r4/Concat  num_inputs=2  dbl_ovrd=off  block_type=concat
      settings: block_version=11.3
  Concat1 : xbsIndex_r4/Concat  num_inputs=2  dbl_ovrd=off  block_type=concat
      settings: block_version=11.3
  Convert{,1..3} (4 alike) : xbsIndex_r4/Convert  arith_type="Signed  (2's comp)"  n_bits=24  bin_pt=24 - (bw_bit_width - bw_bin_pt)  quantization=Truncate  overflow=Wrap  en=off  latency=0  dbl_ovrd=off  pipeline=off  block_type=convert
      settings: block_version=11.4
  Reinterpret{1,12,15..16,24..25} (6 alike) : xbsIndex_r4/Reinterpret  force_arith_type=on  arith_type="Signed  (2's comp)"  force_bin_pt=off  bin_pt=0  block_type=reinterpret
      settings: infoedit="Changes signal type without altering the binary representation.   You can changed the signal between signed and unsigned, and relocate the binary point.<br><br>Hardware notes: In hardware this block costs nothing.<br><br>Example:  Suppose the input is 6 bits wide, signed, with 2 fractional bits, and the output is forced to unsigned with 0 fractional bits.  Then an input of -2.0 (1110.00 in binary 2's complement) becomes an output of 56 (111000 in binary)."  block_version=11.3
  Reinterpret{2..4,10} (4 alike) : xbsIndex_r4/Reinterpret  force_arith_type=on  arith_type="Signed  (2's comp)"  force_bin_pt=on  bin_pt=24 - (bw_bit_width - bw_bin_pt)  block_type=reinterpret
      settings: infoedit="Changes signal type without altering the binary representation.   You can changed the signal between signed and unsigned, and relocate the binary point.<br><br>Hardware notes: In hardware this block costs nothing.<br><br>Example:  Suppose the input is 6 bits wide, signed, with 2 fractional bits, and the output is forced to unsigned with 0 fractional bits.  Then an input of -2.0 (1110.00 in binary 2's complement) becomes an output of 56 (111000 in binary)."  block_version=11.3
  Reinterpret{5..8} (4 alike) : xbsIndex_r4/Reinterpret  force_arith_type=on  arith_type=Unsigned  force_bin_pt=on  bin_pt=0  block_type=reinterpret
      settings: infoedit="Changes signal type without altering the binary representation.   You can changed the signal between signed and unsigned, and relocate the binary point.<br><br>Hardware notes: In hardware this block costs nothing.<br><br>Example:  Suppose the input is 6 bits wide, signed, with 2 fractional bits, and the output is forced to unsigned with 0 fractional bits.  Then an input of -2.0 (1110.00 in binary 2's complement) becomes an output of 56 (111000 in binary)."  block_version=11.3
  a1 : xbsIndex_r4/Slice  nbits=30  boolean_output=off  mode=Upper Bit Location + Width  bit1=0  base1=MSB of Input  bit0=18  base0=LSB of Input  dbl_ovrd=off  block_type=slice
      settings: block_version=11.3
  a5 : xbsIndex_r4/Slice  nbits=30  boolean_output=off  mode=Upper Bit Location + Width  bit1=0  base1=MSB of Input  bit0=18  base0=LSB of Input  dbl_ovrd=off  block_type=slice
      settings: block_version=11.3
  alucode4 : xbsIndex_r4/Constant  arith_type=Unsigned  const=3  n_bits=4  bin_pt=0  explicit_period=on  period=1  equ=P=C  opselect=C  inp2=PCIN>>17  opr=+  inp1=P  carry=CIN  dbl_ovrd=off  block_type=constant
  alucode8 : xbsIndex_r4/Constant  arith_type=Unsigned  const=0  n_bits=4  bin_pt=0  explicit_period=on  period=1  equ=P=C  opselect=C  inp2=PCIN>>17  opr=+  inp1=P  carry=CIN  dbl_ovrd=off  block_type=constant
  ambw : xbsIndex_r4/DSP48E  use_a=Direct from A Port  use_b=Direct from B Port  reset_preg=off  pattern_from_creg=off  pattern='000000000000'  mask_from_creg=off  pattern_mask='3FFFFFFFFFFF'  sel_rounding_mask=Select mask  use_op=off  use_creg=on  rst_all=off  en_all=off  use_pcin=off  use_carrycascin=off  use_multsignin=off  use_carryout=off  use_patterndetect=off  use_patternbdetect=off  use_overflow=off  use_underflow=off  use_acout=off  use_bcout=off  use_pcout=off  use_multsignout=off  use_carrycascout=off  pipeline_a=1  pipeline_b=1  pipeline_acout=1  pipeline_bcout=1  pipeline_c=on  pipeline_p=on  pipeline_mult=on  pipeline_opmode=on  pipeline_alumode=on  pipeline_carryin=on  pipeline_carryinsel=on  rst_a=off  rst_b=off  rst_c=off  rst_mult=off  rst_p=off  rst_carry_in=off  rst_alumode=off  rst_ctrl=off  en_a1=off  en_a2=off  en_b1=off  en_b2=off  en_c=off  en_mult=off  en_p=off  en_carry_in=off  en_alumode=off  en_multcarryin=off  en_ctrl=off  use_synth_model=off  addsub_mode=TWO24  xl_useadderonly=off  block_type=dsp48e
      settings: block_version=10.1.3
  apbw : xbsIndex_r4/DSP48E  use_a=Direct from A Port  use_b=Direct from B Port  reset_preg=off  pattern_from_creg=off  pattern='000000000000'  mask_from_creg=off  pattern_mask='3FFFFFFFFFFF'  sel_rounding_mask=Select mask  use_op=off  use_creg=on  rst_all=off  en_all=off  use_pcin=off  use_carrycascin=off  use_multsignin=off  use_carryout=off  use_patterndetect=off  use_patternbdetect=off  use_overflow=off  use_underflow=off  use_acout=off  use_bcout=off  use_pcout=off  use_multsignout=off  use_carrycascout=off  pipeline_a=1  pipeline_b=1  pipeline_acout=1  pipeline_bcout=1  pipeline_c=on  pipeline_p=on  pipeline_mult=on  pipeline_opmode=on  pipeline_alumode=on  pipeline_carryin=on  pipeline_carryinsel=on  rst_a=off  rst_b=off  rst_c=off  rst_mult=off  rst_p=off  rst_carry_in=off  rst_alumode=off  rst_ctrl=off  en_a1=off  en_a2=off  en_b1=off  en_b2=off  en_c=off  en_mult=off  en_p=off  en_carry_in=off  en_alumode=off  en_multcarryin=off  en_ctrl=off  use_synth_model=off  addsub_mode=TWO24  xl_useadderonly=off  block_type=dsp48e
      settings: block_version=10.1.3
  apbw_re_slice : xbsIndex_r4/Slice  nbits=24  boolean_output=off  mode=Lower Bit Location + Width  bit1=0  base1=MSB of Input  bit0=0  base0=LSB of Input  dbl_ovrd=off  block_type=slice
      settings: block_version=11.3
  apbw_re_slice1 : xbsIndex_r4/Slice  nbits=24  boolean_output=off  mode=Upper Bit Location + Width  bit1=0  base1=MSB of Input  bit0=24  base0=LSB of Input  dbl_ovrd=off  block_type=slice
      settings: block_version=11.3
  apbw_re_slice2 : xbsIndex_r4/Slice  nbits=24  boolean_output=off  mode=Upper Bit Location + Width  bit1=0  base1=MSB of Input  bit0=24  base0=LSB of Input  dbl_ovrd=off  block_type=slice
      settings: block_version=11.3
  apbw_re_slice3 : xbsIndex_r4/Slice  nbits=24  boolean_output=off  mode=Lower Bit Location + Width  bit1=0  base1=MSB of Input  bit0=0  base0=LSB of Input  dbl_ovrd=off  block_type=slice
      settings: block_version=11.3
  b1 : xbsIndex_r4/Slice  nbits=18  boolean_output=off  mode=Lower Bit Location + Width  bit1=0  base1=MSB of Input  bit0=0  base0=LSB of Input  dbl_ovrd=off  block_type=slice
      settings: block_version=11.3
  b5 : xbsIndex_r4/Slice  nbits=18  boolean_output=off  mode=Lower Bit Location + Width  bit1=0  base1=MSB of Input  bit0=0  base0=LSB of Input  dbl_ovrd=off  block_type=slice
      settings: block_version=11.3
  carryin4 : xbsIndex_r4/Constant  arith_type=Unsigned  const=0  n_bits=1  bin_pt=0  explicit_period=on  period=1  equ=P=C  opselect=C  inp2=PCIN>>17  opr=+  inp1=P  carry=CIN  dbl_ovrd=off  block_type=constant
  carryin8 : xbsIndex_r4/Constant  arith_type=Unsigned  const=0  n_bits=1  bin_pt=0  explicit_period=on  period=1  equ=P=C  opselect=C  inp2=PCIN>>17  opr=+  inp1=P  carry=CIN  dbl_ovrd=off  block_type=constant
  carryinsel4 : xbsIndex_r4/Constant  arith_type=Unsigned  const=0  n_bits=3  bin_pt=0  explicit_period=on  period=1  equ=P=C  opselect=C  inp2=PCIN>>17  opr=+  inp1=P  carry=CIN  dbl_ovrd=off  block_type=constant
  carryinsel8 : xbsIndex_r4/Constant  arith_type=Unsigned  const=0  n_bits=3  bin_pt=0  explicit_period=on  period=1  equ=P=C  opselect=C  inp2=PCIN>>17  opr=+  inp1=P  carry=CIN  dbl_ovrd=off  block_type=constant
  opcode4 : xbsIndex_r4/Constant  arith_type=Unsigned  const=51  n_bits=7  bin_pt=0  explicit_period=on  period=1  equ=P=C  opselect=C  inp2=PCIN>>17  opr=+  inp1=P  carry=CIN  dbl_ovrd=off  block_type=constant
  opcode8 : xbsIndex_r4/Constant  arith_type=Unsigned  const=15  n_bits=7  bin_pt=0  explicit_period=on  period=1  equ=P=C  opselect=C  inp2=PCIN>>17  opr=+  inp1=P  carry=CIN  dbl_ovrd=off  block_type=constant
  a+bw_re : Outport
  a+bw_im : Outport  Port=2
  a-bw_re : Outport  Port=3
  a-bw_im : Outport  Port=4
  wires:
  Reinterpret8/1 -> Concat1/2
  Reinterpret7/1 -> Concat1/1
  Reinterpret6/1 -> Concat/2
  Reinterpret5/1 -> Concat/1
  Convert3/1 -> Reinterpret8/1
  Convert2/1 -> Reinterpret7/1
  Convert1/1 -> Reinterpret6/1
  Convert/1 -> Reinterpret5/1
  Reinterpret4/1 -> a-bw_im/1
  Reinterpret3/1 -> a-bw_re/1
  Reinterpret2/1 -> a+bw_im/1
  Reinterpret12/1 -> ambw/3
  apbw_re_slice3/1 -> Reinterpret4/1
  ambw/1 -> apbw_re_slice2/1, apbw_re_slice3/1
  carryinsel4/1 -> ambw/7
  carryin4/1 -> ambw/6
  alucode4/1 -> ambw/5
  opcode4/1 -> ambw/4
  Reinterpret16/1 -> ambw/2
  b1/1 -> Reinterpret16/1
  Reinterpret15/1 -> ambw/1
  a1/1 -> Reinterpret15/1
  apbw_re_slice2/1 -> Reinterpret3/1
  Reinterpret10/1 -> a+bw_re/1
  Reinterpret1/1 -> apbw/3
  apbw_re_slice/1 -> Reinterpret2/1
  apbw/1 -> apbw_re_slice1/1, apbw_re_slice/1
  carryinsel8/1 -> apbw/7
  carryin8/1 -> apbw/6
  alucode8/1 -> apbw/5
  opcode8/1 -> apbw/4
  Reinterpret25/1 -> apbw/2
  b5/1 -> Reinterpret25/1
  Reinterpret24/1 -> apbw/1
  a5/1 -> Reinterpret24/1
  apbw_re_slice1/1 -> Reinterpret10/1
  Concat1/1 -> a1/1, b1/1, Reinterpret1/1
  Concat/1 -> b5/1, a5/1, Reinterpret12/1
  bw_im/1 -> Convert3/1
  bw_re/1 -> Convert2/1
  a_im/1 -> Convert1/1
  a_re/1 -> Convert/1

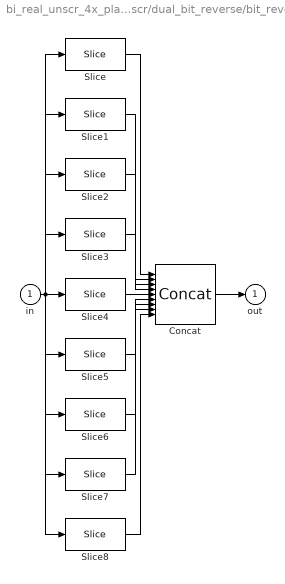
== system bi_real_unscr_4x_plan/biplex_4x_unscr/dual_bit_reverse/bit_reverse ==
  in : Inport
  Concat : xbsIndex_r4/Concat  num_inputs=9  dbl_ovrd=off  block_type=concat
  Slice : xbsIndex_r4/Slice  nbits=1  boolean_output=off  mode=Lower Bit Location + Width  bit1=0  base1=MSB of Input  bit0=0  base0=MSB of Input  dbl_ovrd=off  block_type=slice
  Slice1 : xbsIndex_r4/Slice  nbits=1  boolean_output=off  mode=Lower Bit Location + Width  bit1=1  base1=MSB of Input  bit0=0  base0=MSB of Input  dbl_ovrd=off  block_type=slice
  Slice2 : xbsIndex_r4/Slice  nbits=1  boolean_output=off  mode=Lower Bit Location + Width  bit1=2  base1=MSB of Input  bit0=0  base0=MSB of Input  dbl_ovrd=off  block_type=slice
  Slice3 : xbsIndex_r4/Slice  nbits=1  boolean_output=off  mode=Lower Bit Location + Width  bit1=3  base1=MSB of Input  bit0=0  base0=MSB of Input  dbl_ovrd=off  block_type=slice
  Slice4 : xbsIndex_r4/Slice  nbits=1  boolean_output=off  mode=Lower Bit Location + Width  bit1=4  base1=MSB of Input  bit0=0  base0=MSB of Input  dbl_ovrd=off  block_type=slice
  Slice5 : xbsIndex_r4/Slice  nbits=1  boolean_output=off  mode=Lower Bit Location + Width  bit1=5  base1=MSB of Input  bit0=0  base0=MSB of Input  dbl_ovrd=off  block_type=slice
  Slice6 : xbsIndex_r4/Slice  nbits=1  boolean_output=off  mode=Lower Bit Location + Width  bit1=6  base1=MSB of Input  bit0=0  base0=MSB of Input  dbl_ovrd=off  block_type=slice
  Slice7 : xbsIndex_r4/Slice  nbits=1  boolean_output=off  mode=Lower Bit Location + Width  bit1=7  base1=MSB of Input  bit0=0  base0=MSB of Input  dbl_ovrd=off  block_type=slice
  Slice8 : xbsIndex_r4/Slice  nbits=1  boolean_output=off  mode=Lower Bit Location + Width  bit1=8  base1=MSB of Input  bit0=0  base0=MSB of Input  dbl_ovrd=off  block_type=slice
  out : Outport
  wires:
  Slice/1 -> Concat/1
  Slice1/1 -> Concat/2
  Slice2/1 -> Concat/3
  Slice3/1 -> Concat/4
  Slice4/1 -> Concat/5
  Slice5/1 -> Concat/6
  Slice6/1 -> Concat/7
  Slice7/1 -> Concat/8
  Slice8/1 -> Concat/9
  Concat/1 -> out/1
  in/1 -> Slice/1, Slice1/1, Slice2/1, Slice3/1, Slice4/1, Slice5/1, Slice6/1, Slice7/1, Slice8/1

== system bi_real_unscr_4x_plan/biplex_4x_unscr/dual_bit_reverse/bit_reverse1 ==
  in : Inport
  Concat : xbsIndex_r4/Concat  num_inputs=9  dbl_ovrd=off  block_type=concat
  Slice : xbsIndex_r4/Slice  nbits=1  boolean_output=off  mode=Lower Bit Location + Width  bit1=0  base1=MSB of Input  bit0=0  base0=MSB of Input  dbl_ovrd=off  block_type=slice
  Slice1 : xbsIndex_r4/Slice  nbits=1  boolean_output=off  mode=Lower Bit Location + Width  bit1=1  base1=MSB of Input  bit0=0  base0=MSB of Input  dbl_ovrd=off  block_type=slice
  Slice2 : xbsIndex_r4/Slice  nbits=1  boolean_output=off  mode=Lower Bit Location + Width  bit1=2  base1=MSB of Input  bit0=0  base0=MSB of Input  dbl_ovrd=off  block_type=slice
  Slice3 : xbsIndex_r4/Slice  nbits=1  boolean_output=off  mode=Lower Bit Location + Width  bit1=3  base1=MSB of Input  bit0=0  base0=MSB of Input  dbl_ovrd=off  block_type=slice
  Slice4 : xbsIndex_r4/Slice  nbits=1  boolean_output=off  mode=Lower Bit Location + Width  bit1=4  base1=MSB of Input  bit0=0  base0=MSB of Input  dbl_ovrd=off  block_type=slice
  Slice5 : xbsIndex_r4/Slice  nbits=1  boolean_output=off  mode=Lower Bit Location + Width  bit1=5  base1=MSB of Input  bit0=0  base0=MSB of Input  dbl_ovrd=off  block_type=slice
  Slice6 : xbsIndex_r4/Slice  nbits=1  boolean_output=off  mode=Lower Bit Location + Width  bit1=6  base1=MSB of Input  bit0=0  base0=MSB of Input  dbl_ovrd=off  block_type=slice
  Slice7 : xbsIndex_r4/Slice  nbits=1  boolean_output=off  mode=Lower Bit Location + Width  bit1=7  base1=MSB of Input  bit0=0  base0=MSB of Input  dbl_ovrd=off  block_type=slice
  Slice8 : xbsIndex_r4/Slice  nbits=1  boolean_output=off  mode=Lower Bit Location + Width  bit1=8  base1=MSB of Input  bit0=0  base0=MSB of Input  dbl_ovrd=off  block_type=slice
  out : Outport
  wires:
  in/1 -> Slice8/1, Slice7/1, Slice6/1, Slice5/1, Slice4/1, Slice3/1, Slice2/1, Slice1/1, Slice/1
  Concat/1 -> out/1
  Slice8/1 -> Concat/9
  Slice7/1 -> Concat/8
  Slice6/1 -> Concat/7
  Slice5/1 -> Concat/6
  Slice4/1 -> Concat/5
  Slice3/1 -> Concat/4
  Slice2/1 -> Concat/3
  Slice1/1 -> Concat/2
  Slice/1 -> Concat/1
